simulink model "Subject3"  (R2022b)
settings: Solver=VariableStepAuto  StartTime=0.0  StopTime=10  RelTol=1e-3
libraries: simulink x1, mpcadaslib x1
settings Model: Creator=ParkJunHo  LastModifiedBy=ParkJunHo

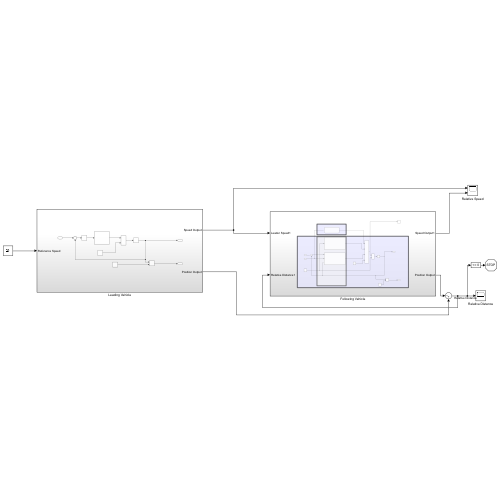
[thumbnail: Simulink's stored preview of the top-level diagram]
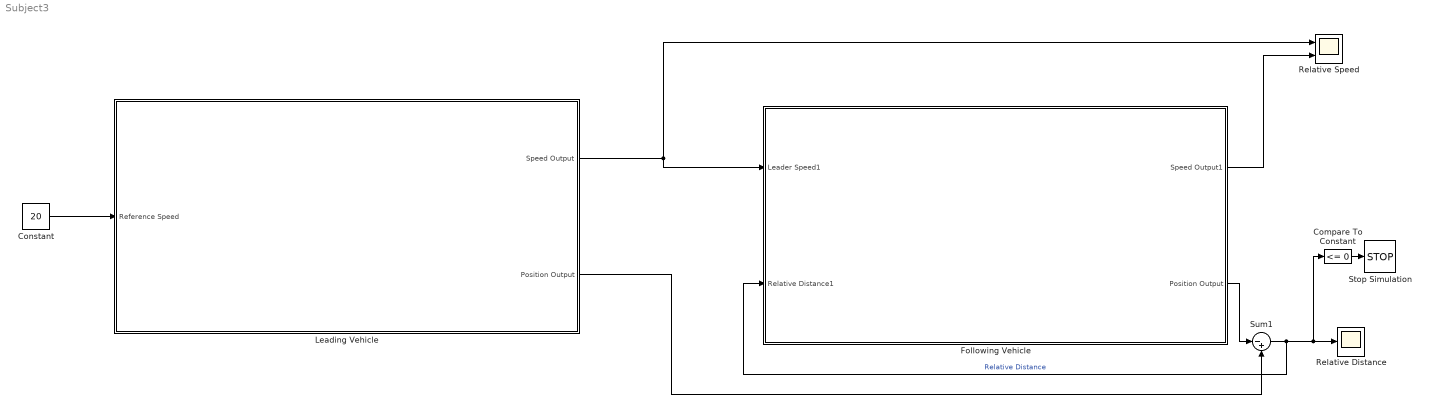
== system Subject3 ==
  Compare To Constant : simulink/Logic and Bit Operations/Compare To Constant  relop=<=  const=0  OutDataTypeStr=boolean
  Constant : Constant  Value=20
  Following Vehicle : Subsystem
  Leading Vehicle : Subsystem
  Relative Distance : Scope
  Relative Speed : Scope  NumInputPorts=2
  Stop Simulation : Stop
  Sum1 : Sum  Inputs=|-+
  wires:
  Constant/1 -> Leading Vehicle/1(Reference Speed)
  Leading Vehicle/1(Speed Output) -> Relative Speed/1, Following Vehicle/1(Leader Speed1)
  Leading Vehicle/2(Position Output) -> Sum1/2
  Sum1/1 -> Following Vehicle/2(Relative Distance1), Compare To Constant/1, Relative Distance/1  "Relative Distance"
  Compare To Constant/1 -> Stop Simulation/1
  Following Vehicle/1(Speed Output1) -> Relative Speed/2
  Following Vehicle/2(Position Output) -> Sum1/1

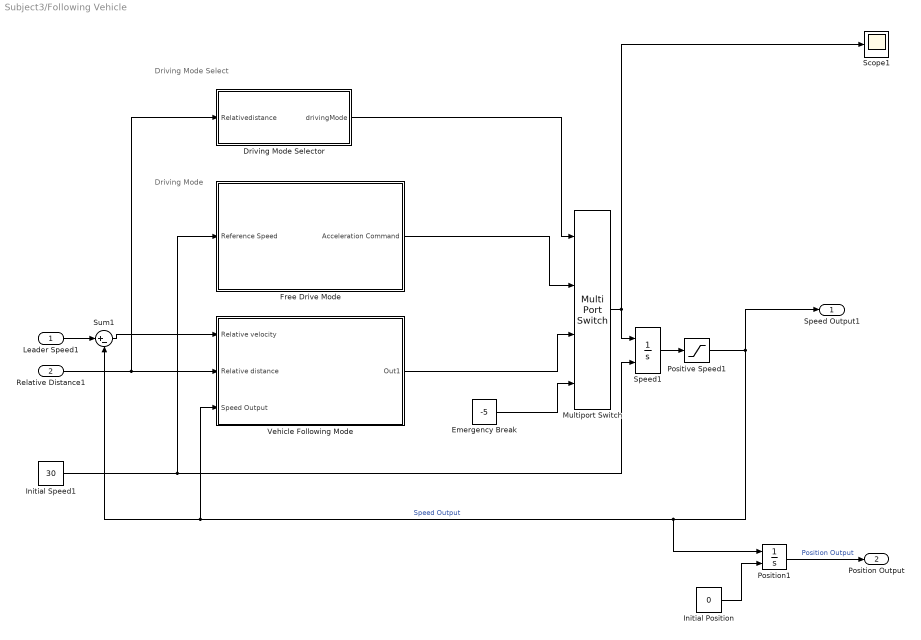
== system Subject3/Following Vehicle ==
  note: Driving Mode
  note: Driving Mode Select
  Leader Speed1 : Inport
  Relative Distance1 : Inport  Port=2
  Driving Mode Selector : Stateflow chart  TreatAsAtomicUnit=on
  Emergency Break : Constant  Value=-5
  Free Drive Mode : Subsystem
  Initial Position : Constant  Value=0
  Initial Speed1 : Constant  Value=30
  Multiport Switch : MultiPortSwitch  SaturateOnIntegerOverflow=off  InputSameDT=off
  Position1 : Integrator  InitialConditionSource=external
  Positive Speed1 : Saturate  UpperLimit=inf  LowerLimit=0
  Scope1 : Scope
  Speed1 : Integrator  InitialConditionSource=external
  Sum1 : Sum  Inputs=|+-
  Vehicle Following Mode : Subsystem
  Speed Output1 : Outport
  Position Output : Outport  Port=2
  wires:
  Multiport Switch/1 -> Scope1/1, Speed1/1
  Vehicle Following Mode/1(Out1) -> Multiport Switch/3
  Driving Mode Selector/1(drivingMode) -> Multiport Switch/1
  Emergency Break/1 -> Multiport Switch/4
  Speed1/1 -> Positive Speed1/1
  Position1/1 -> Position Output/1  "Position Output"
  Positive Speed1/1 -> Speed Output1/1, Position1/1, Vehicle Following Mode/3(Speed Output), Sum1/2  "Speed Output"
  Sum1/1 -> Vehicle Following Mode/1(Relative velocity)
  Free Drive Mode/1(Acceleration Command) -> Multiport Switch/2
  Relative Distance1/1 -> Vehicle Following Mode/2(Relative distance), Driving Mode Selector/1(Relativedistance)
  Leader Speed1/1 -> Sum1/1
  Initial Position/1 -> Position1/2
  Initial Speed1/1 -> Free Drive Mode/1(Reference Speed), Speed1/2

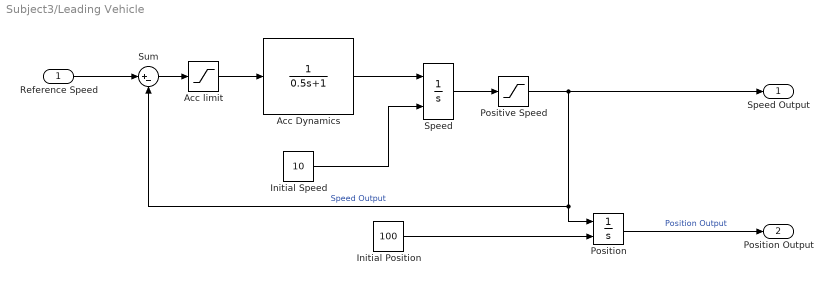
== system Subject3/Leading Vehicle ==
  Reference Speed : Inport
  Acc Dynamics : TransferFcn  Denominator=[0.5 1]
  Acc limit : Saturate  UpperLimit=2  LowerLimit=-3
  Initial Position : Constant  Value=100
  Initial Speed : Constant  Value=10
  Position : Integrator  InitialConditionSource=external
  Positive Speed : Saturate  UpperLimit=inf  LowerLimit=0
  Speed : Integrator  InitialConditionSource=external
  Sum : Sum  Inputs=|+-
  Speed Output : Outport
  Position Output : Outport  Port=2
  wires:
  Sum/1 -> Acc limit/1
  Positive Speed/1 -> Speed Output/1, Position/1, Sum/2  "Speed Output"
  Speed/1 -> Positive Speed/1
  Position/1 -> Position Output/1  "Position Output"
  Acc Dynamics/1 -> Speed/1
  Initial Position/1 -> Position/2
  Acc limit/1 -> Acc Dynamics/1
  Initial Speed/1 -> Speed/2
  Reference Speed/1 -> Sum/1

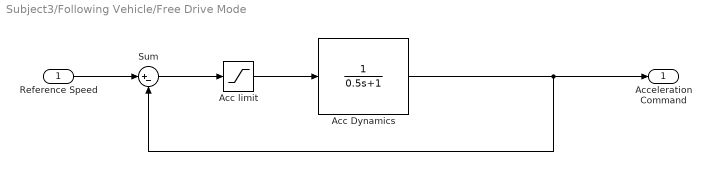
== system Subject3/Following Vehicle/Free Drive Mode ==
  Reference Speed : Inport
  Acc Dynamics : TransferFcn  Denominator=[0.5 1]
  Acc limit : Saturate  UpperLimit=2  LowerLimit=-3
  Sum : Sum  Inputs=|+-
  Acceleration Command : Outport
  wires:
  Acc Dynamics/1 -> Sum/2, Acceleration Command/1
  Acc limit/1 -> Acc Dynamics/1
  Reference Speed/1 -> Sum/1
  Sum/1 -> Acc limit/1

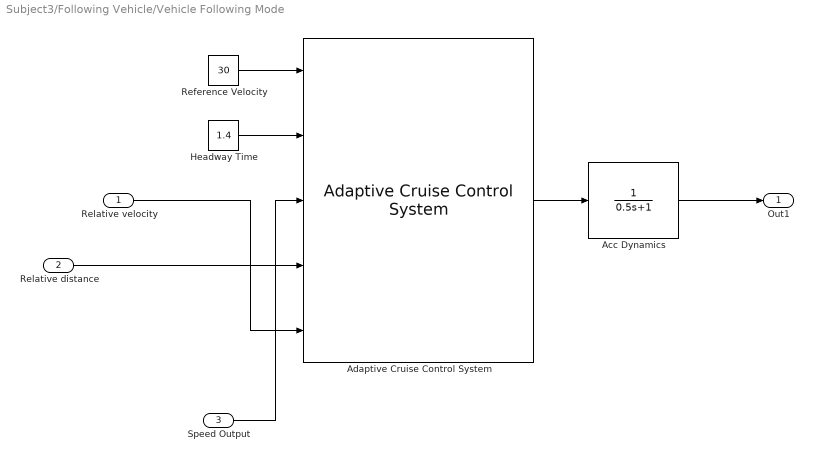
== system Subject3/Following Vehicle/Vehicle Following Mode ==
  Relative velocity : Inport
  Relative distance : Inport  Port=2
  Speed Output : Inport  Port=3
  Acc Dynamics : TransferFcn  Denominator=[0.5 1]
  Adaptive Cruise Control System : mpcadaslib/Adaptive Cruise Control System  EgoModel=tf(1,[0.5,1,0])  InitialEgoVelocity=30  DefaultSpacing=10  MaxVelocity=50  MinAcceleration=-3  amin_ext=off  MaxAcceleration=2  amax_ext=off  Ts=0.5  PredictionHorizon=200  ControllerBehavior=0.590  suboptimal=off  maxiter=10  datatypeopt=double  optmode=off  trackmode=off
      settings: LibrarySourceBlock=mpclib/Automated Driving/Adaptive Cruise Control System
  Headway Time : Constant  Value=1.4
  Reference Velocity : Constant  Value=30
  Out1 : Outport
  wires:
  Relative distance/1 -> Adaptive Cruise Control System/4
  Headway Time/1 -> Adaptive Cruise Control System/2
  Adaptive Cruise Control System/1 -> Acc Dynamics/1
  Reference Velocity/1 -> Adaptive Cruise Control System/1
  Speed Output/1 -> Adaptive Cruise Control System/3
  Acc Dynamics/1 -> Out1/1
  Relative velocity/1 -> Adaptive Cruise Control System/5

== stateflow chart Subject3/Following Vehicle/Driving Mode Selector ==
  state FreeDrive
    entry:
    drivingMode=1;
  state VehicleFollowing
    entry:
    drivingMode=2;
  state EmergencyBrake
    entry:
    drivingMode=3;
  (default) -> FreeDrive
  VehicleFollowing -> FreeDrive [order 1] : [Relativedistance>60]
  FreeDrive -> VehicleFollowing [order 1] : [Relativedistance<=60]
  FreeDrive -> EmergencyBrake [order 2] : [Relativedistance<=30]
  VehicleFollowing -> EmergencyBrake [order 2] : [Relativedistance<=30]
  EmergencyBrake -> VehicleFollowing : [Relativedistance>60]
  data: Relativedistance input; drivingMode output
